simulink library "libc_control_pressure"  (R2015b)
settings: Solver=FixedStepDiscrete  StartTime=0.0  StopTime=Inf  FixedStep=0.004  RelTol=1e-3
PostLoadFcn:
  | , if any(exist('dsrtsu_mdlpostloadfcn', 'file') == [2, 3, 6]), try dsrtsu_mdlpostloadfcn('Execute', bdroot); catch fprintf('Error in PostLoadFcn (dsrtsu_mdlpostloadfcn) for model "%s":\n %s\n', bdroot, lasterr); end, end,
undefined symbols (not defined in the file or in its folder): CONST, den, DiscIntNeverNeededParam, num, p1i, tA
libraries: simulink x21, libc_parts_valves x17, libc_filters_diff x9, libbha_parts_bellows x4, libc_parts_tubes x2, PMC_lib x1
(part 1 of 2)
settings Model: DSRTSU_INTERNAL_RTI_VER=470  DSRTSU_INTERNAL_RTI_TYPE=rti1007  DSRTSU_INTERNAL_RTIFPGA=60  Creator=Falkenhahn  LastModifiedBy=Falkenhahn
settings DataIOCC: SaveFormat=Array
settings OptimizationCC: BlockReduction=off  OptimizeBlockIOStorage=off  BufferReuse=off  GlobalBufferReuse=off  ExpressionFolding=off  LocalBlockOutputs=off
settings DebuggingCC: UnderspecifiedInitializationDetection=Classic  MergeDetectMultiDrivingBlocksExec=none  SolverPrmCheckMsg=warning
settings HardwareCC: ProdBitPerPointer=32  ProdLargestAtomicFloat=None  ProdEndianess=BigEndian  ProdWordSize=32  ProdHWDeviceType=Generic->Custom  TargetIntDivRoundTo=Zero  TargetEndianess=BigEndian  TargetHWDeviceType=Generic->Custom
settings RTWCC: SystemTargetFile=rti1007.tlc  MakeCommand=make_rti  TemplateMakefile=rti1007.tmf  Description=dSPACE DS1007 Hardware Platform
settings STFCustomTargetCC: ParMdlRefBuildCompliant=on  ConcurrentExecutionCompliant=off  MatFileLogging=on  SystemTargetFile=rti1007.tlc
settings GRTTargetCC: CompOptLevelCompliant=off  ConcurrentExecutionCompliant=off  GeneratePreprocessorConditionals=Disable all  CombineOutputUpdateFcns=off  GRTInterface=on  UseToolchainInfoCompliant=off  ExtModeMexFile=noextcomm
settings ConfigComp: CovModelRefEnable=Off

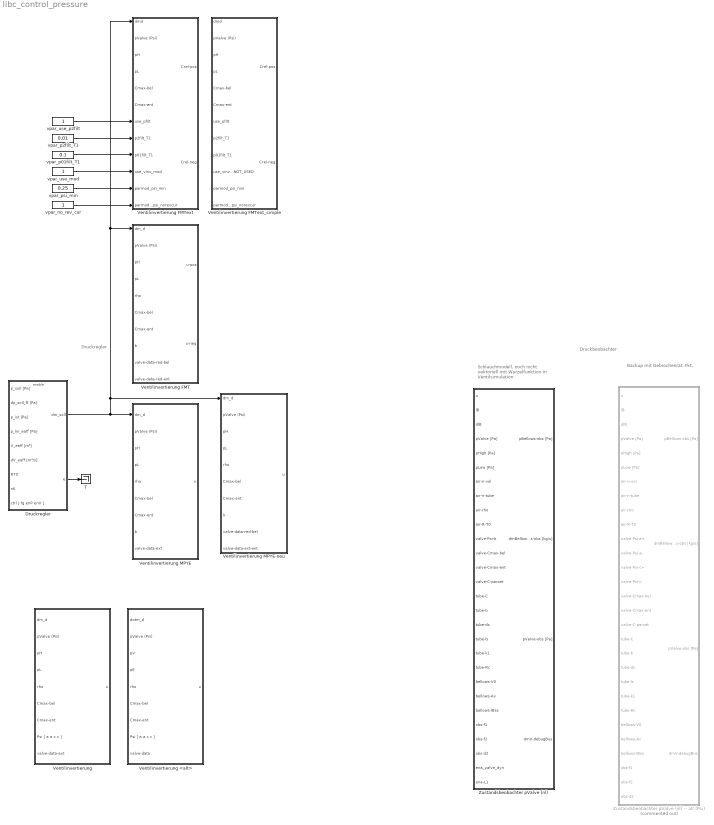
== system libc_control_pressure ==
  note: Backup mit Gebrochenrat. Fkt.
  note: Schlauchmodell, noch nicht vektoriell
      | mit Wurzelfunktion in Ventilsimulation
  note: Druckregler
  note: Druckbeobachter
  Druckregler : Subsystem
  T : Terminator
  Ventilinvertierung : Subsystem
      settings: AttributesFormatString=uses local sample time tA
  Ventilinvertierung <alt> : Subsystem
      settings: AttributesFormatString=uses local sample time tA
  Ventilinvertierung FMT : Subsystem
  Ventilinvertierung FMText : Subsystem
      settings: RTWFcnNameOpts=Use subsystem name  RTWFileNameOpts=Use function name
  Ventilinvertierung FMText_simple : Subsystem
      settings: RTWFcnNameOpts=Use subsystem name  RTWFileNameOpts=Use function name
  Ventilinvertierung MPYE : Subsystem
      settings: AttributesFormatString=uses local sample time tA
  Ventilinvertierung MPYE-neu : Subsystem
  Zustandsbeobachter pValve (nl) : Subsystem
  "Zustandsbeobachter pValve (nl) -- alt (Psi)" : Subsystem  Commented=on
  vpar_no_rev_cur : Constant
      settings: AttributesFormatString=|
      | Filterung des Kammerdrucks
      | bei FMT-Ventilen. Schnelle
      | Sprünge können eh nicht
      | kompensiert werden, da
      | Ventildynamik zu langsam
  vpar_p01filt_T1 : Constant  Value=0.1
  vpar_p2filt_T1 : Constant  Value=0.01
  vpar_psi_min : Constant  Value=0.25
  vpar_use_mod : Constant
  vpar_use_p2filt : Constant
  wires:
  Druckregler/2(e) -> T/1
  Druckregler/1(dm_soll) -> Ventilinvertierung MPYE-neu/1(dm_d), Ventilinvertierung FMT/1(dm_d), Ventilinvertierung FMText/1(dmd), Ventilinvertierung MPYE/1(dm_d)
  vpar_no_rev_cur/1 -> Ventilinvertierung FMText/12(parmod_psi_norevcur)
  vpar_psi_min/1 -> Ventilinvertierung FMText/11(parmod_psi_min)
  vpar_use_mod/1 -> Ventilinvertierung FMText/10(use_vinv_mod)
  vpar_p2filt_T1/1 -> Ventilinvertierung FMText/8(p2filt_T1)
  vpar_use_p2filt/1 -> Ventilinvertierung FMText/7(use_pfilt)
  vpar_p01filt_T1/1 -> Ventilinvertierung FMText/9(p01filt_T1)

== system libc_control_pressure/Druckregler ==
  note: Allgemeiner Druckregler (basierend auf dem
      | Druckregler von Alexander Hildebrandt | hild)
      |
      | Eingänge:
      | Drücke (alle in [Pa] absolut):
      | Solldruck, Solldruckänderung, Istdruck, Linearisierungsdruck
      | Volumen und Volumenänderung
      | Produkt RT0 und Polytropenkoeffizient nK
      | Reglerparameter ctrl
      |
      | Ausgang: Sollmassenstrom dm [kg/s] für Ventilinvertierung
  note: Funktionsbeschreibung
  note: Linearisierungsdruck p_lin_eaff kann entweder mit
      | Solldruck (zur Feedforward-Linearisierung) oder mit
      | Istdruck (zur Zustandslinearisierung) verwendet werden,
      | um Volumenänderungen dV =/= 0 zu kompensieren. Entsprechend
      | sollte dann auch die Volumenberechnung mittels Soll- oder Istgrößen geschehen
  note: Linearisierungsdruck
  note: Beschreibung der Parameter des Konfigurationseingangs ctrl
      | (*) empfohlener Wert
      |
      | fg [Hz]: Grenzfrequenz (*4Hz)
      | enP {0|1*}: aktiviere P-Regler
      | enV {0|1*}: aktiviere Vorsteuerung
  note: Reglerparameter "ctrl"
  p_soll [Pa] : Inport
  dp_soll_ff [Pa] : Inport  Port=2
  p_ist [Pa] : Inport  Port=3
  p_lin_eaff [Pa] : Inport  Port=4
  V_eaff [m³] : Inport  Port=5
  dV_eaff [m³/s] : Inport  Port=6
  RT0 : Inport  Port=7
  nK : Inport  Port=8
  ctrl [ fg enP enV ] : Inport  Port=9
  Enable : EnablePort  StatesWhenEnabling=reset
      settings: AttributesFormatString=%<StatesWhenEnabling> states\nwhen enabling
  Drucklinearsierung : Subsystem
  Folgeregler : Subsystem
  dm_soll : Outport
  e : Outport  Port=2
  wires:
  nK/1 -> Drucklinearsierung/7(nK)
  p_ist [Pa]/1 -> Folgeregler/3(p_ist)
  RT0/1 -> Drucklinearsierung/6(RT0)
  ctrl [ fg enP enV ]/1 -> Folgeregler/4(ctrl [ fgP enP enV ])
  p_lin_eaff [Pa]/1 -> Drucklinearsierung/5(p (E/A))
  dV_eaff [m³/s]/1 -> Drucklinearsierung/4(dV)
  V_eaff [m³]/1 -> Drucklinearsierung/3(V)
  Folgeregler/1(e) -> e/1
  p_soll [Pa]/1 -> Folgeregler/1(p_soll)
  dp_soll_ff [Pa]/1 -> Folgeregler/2(dp_soll)
  Folgeregler/3(nu_Vst) -> Drucklinearsierung/2(nu_in_Vorst)
  Folgeregler/2(nu_P) -> Drucklinearsierung/1(nu_in_PReg)
  Drucklinearsierung/1(dm) -> dm_soll/1

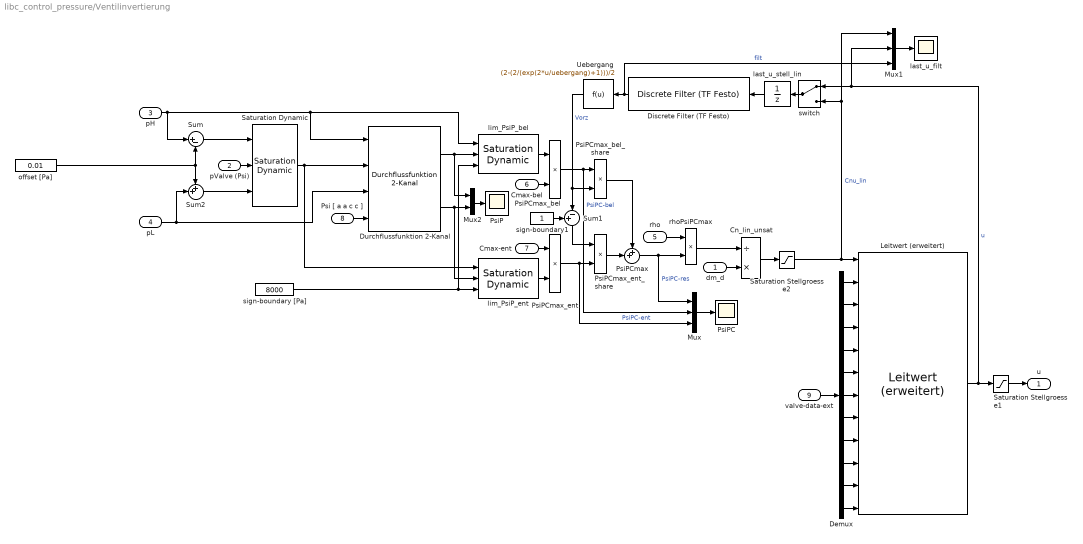
== system libc_control_pressure/Ventilinvertierung ==
  dm_d : Inport
  pValve (Psi) : Inport  Port=2
  pH : Inport  Port=3
  pL : Inport  Port=4
  rho : Inport  Port=5
  Cmax-bel : Inport  Port=6
  Cmax-ent : Inport  Port=7
  Psi [ a a c c ] : Inport  Port=8
  valve-data-ext : Inport  Port=9
  Cn_lin_unsat : Product  Inputs=/*
  Demux : Demux  Outputs=11
  Discrete Filter (TF Festo) : libc_filters_diff/Discrete Filter (TF Festo)  num_a=[1]  den_a=[1/(2*pi*3), 1]  Tsamp=tA  method='ramp'  dar='z'
      settings: AttributesFormatString=|
      | sample time: %<Tsamp> (3Hz)
      | Erhöhung der Eckfrequenz bringt keine
      | sichtbare Performanceverbesserung,
      | nur das Ventilknattern wird lauter.
  Durchflussfunktion 2-Kanal : libc_parts_valves/Durchflussfunktion 2-Kanal
      settings: AttributesFormatString=gebrochenrational
  Leitwert (erweitert) : libc_parts_valves/Leitwert (erweitert)  invertcomp=on
      settings: AttributesFormatString=|
      | inv: Cn --> u (on)
      | hin: u --> Cn (off)
      | Invertiert: %<invertcomp>
  Mux : Mux  Inputs=3
  Mux1 : Mux  Inputs=3
  Mux2 : Mux  Inputs=2
  PsiP : Scope
  PsiPC : Scope
  PsiPCmax : Sum  Inputs=++|
  PsiPCmax_bel : Product
  PsiPCmax_bel_share : Product
  PsiPCmax_ent : Product
  PsiPCmax_ent_share : Product
  Saturation Dynamic : simulink/Discontinuities/Saturation Dynamic  OutMin=[]  OutMax=[]  OutDataTypeStr=Inherit: Same as second input  OutDataType=fixdt(1, 16)  OutScaling=2^-10  DoSatur=off
  Saturation Stellgroesse1 : Saturate  UpperLimit=1  LowerLimit=-1
  Saturation Stellgroesse2 : Saturate  UpperLimit=1  LowerLimit=-1
  Sum : Sum  Inputs=|+-
  Sum1 : Sum  Inputs=+-|
  Sum2 : Sum  Inputs=++|
  Uebergang : Fcn  Expr=(2-(2/(exp(2*u/uebergang)+1)))/2  mask{uebergang=0.1}
      mask prompts: uebergang "Bereich der sanften Umschaltung"
      mask init:
      | u=-1:uebergang:1;
      | y=(tanh(u/uebergang)+1)/2;
      settings: AttributesFormatString=|
      | Weichheit des
      | Übergangs
      | testen (0.1)
      mask Display: plot(u,y)
  last_u_filt : Scope
  last_u_stell_lin : UnitDelay  SampleTime=-1
  lim_PsiP_bel : simulink/Discontinuities/Saturation Dynamic  OutMin=[]  OutMax=[]  OutDataTypeStr=Inherit: Same as second input  OutDataType=fixdt(1, 16)  OutScaling=2^-10  DoSatur=off
  lim_PsiP_ent : simulink/Discontinuities/Saturation Dynamic  OutMin=[]  OutMax=[]  OutDataTypeStr=Inherit: Same as second input  OutDataType=fixdt(1, 16)  OutScaling=2^-10  DoSatur=off
      settings: AttributesFormatString=|
      | PsiP ist immer positiv.
      | PsiP-bel wird durch Kammerdruck
      | beschränkt, nicht durch Entlüftungsdruck
  offset [Pa] : Constant  Value=0.01  SampleTime=tA
      settings: AttributesFormatString=|
      | Num. Offset
      | ca. 0.01 bar als numerische Begrenzung
      | für Psi*P in Randbereichen, damit nicht
      | gegen 0 und Cn_lin_unsat nicht viel zu groß.
      | Jetzt kleiner, da zusätzliche Begrenzung später
      | 
      | sample time: %<SampleTime>
  rhoPsiPCmax : Product  Inputs=**
  sign-boundary [Pa] : Constant  Value=8000
      settings: AttributesFormatString=|
      | untere Grenze für PsiP
      | Da diese Zahl später im Nenner stehen wird, sollte dies etwas größer
      | als 0 sein. Für den numerischen Offset hat sich ein Richtwert von 1000 Pa
      | in der Praxis (untere Grenze) bewährt. Rechnet man dies weiter, kommen
      | für Psi bei pL=1bar, pH=2bar 0.04285 und 0.08065 heraus. PsiP liegt dann bei
      | 8570 und 8146 Pa. Dies lässt sich gut mit 8000Pa abschätzen, sodass der Offset
      | wieder rein numerischer Natur (0.01) sein kann.
      | 
      | Wann wirkt dies: Bei stationären Gleichgewichtslagen (Psi ~0) am Rand des
      | Druckbereichs (nahe Versorgung oder nahe Umgebung) --> Ventil rattert
  sign-boundary1 : Constant
  switch : ManualSwitch
      settings: AttributesFormatString=|
      | da nur Vorzeichen
      | relevant ist, ist es
      | eigentlich egal, ob
      | u oder Cn(u) ver-
      | wendet wird.
      | 
      | Allerdings wirkt
      | Übergang auf u
  u : Outport
  wires:
  rho/1 -> rhoPsiPCmax/1
  Cmax-ent/1 -> PsiPCmax_ent/1
  Cmax-bel/1 -> PsiPCmax_bel/2
  Psi [ a a c c ]/1 -> Durchflussfunktion 2-Kanal/4
  valve-data-ext/1 -> Demux/1
  dm_d/1 -> Cn_lin_unsat/2
  pL/1 -> Sum2/2, Durchflussfunktion 2-Kanal/3
  pValve (Psi)/1 -> Saturation Dynamic/2
  pH/1 -> Sum/1, Durchflussfunktion 2-Kanal/1, lim_PsiP_bel/1
  Mux/1 -> PsiPC/1
  sign-boundary1/1 -> Sum1/1
  Sum1/1 -> PsiPCmax_ent_share/1
  PsiPCmax_ent/1 -> Mux/3, PsiPCmax_ent_share/2  "PsiPC-ent"
  PsiPCmax_bel/1 -> Mux/2, PsiPCmax_bel_share/1  "PsiPC-bel"
  PsiPCmax_bel_share/1 -> PsiPCmax/1
  PsiPCmax_ent_share/1 -> PsiPCmax/2
  Durchflussfunktion 2-Kanal/2 -> lim_PsiP_ent/2, Mux2/2
  Discrete Filter (TF Festo)/1 -> Uebergang/1, Mux1/3  "filt"
  rhoPsiPCmax/1 -> Cn_lin_unsat/1
  PsiPCmax/1 -> Mux/1, rhoPsiPCmax/2  "PsiPC-res"
  lim_PsiP_ent/1 -> PsiPCmax_ent/2
  lim_PsiP_bel/1 -> PsiPCmax_bel/1
  sign-boundary [Pa]/1 -> lim_PsiP_ent/3, lim_PsiP_bel/3
  switch/1 -> last_u_stell_lin/1
  Sum2/1 -> Saturation Dynamic/3
  offset [Pa]/1 -> Sum2/1, Sum/2
  Cn_lin_unsat/1 -> Saturation Stellgroesse2/1
  Durchflussfunktion 2-Kanal/1 -> lim_PsiP_bel/2, Mux2/1
  Saturation Dynamic/1 -> lim_PsiP_ent/1, Durchflussfunktion 2-Kanal/2
  Saturation Stellgroesse2/1 -> Leitwert (erweitert)/1, switch/2, Mux1/1  "Cnu_lin"
  last_u_stell_lin/1 -> Discrete Filter (TF Festo)/1
  Uebergang/1 -> Sum1/2, PsiPCmax_bel_share/2  "Vorz"
  Sum/1 -> Saturation Dynamic/1
  Leitwert (erweitert)/1 -> switch/1, Mux1/2, Saturation Stellgroesse1/1  "u"
  Demux/1 -> Leitwert (erweitert)/2
  Demux/2 -> Leitwert (erweitert)/3
  Demux/3 -> Leitwert (erweitert)/4
  Demux/4 -> Leitwert (erweitert)/5
  Demux/5 -> Leitwert (erweitert)/6
  Demux/6 -> Leitwert (erweitert)/7
  Demux/7 -> Leitwert (erweitert)/8
  Mux1/1 -> last_u_filt/1
  Mux2/1 -> PsiP/1
  Demux/11 -> Leitwert (erweitert)/12
  Demux/9 -> Leitwert (erweitert)/10
  Demux/10 -> Leitwert (erweitert)/11
  Demux/8 -> Leitwert (erweitert)/9
  Saturation Stellgroesse1/1 -> u/1

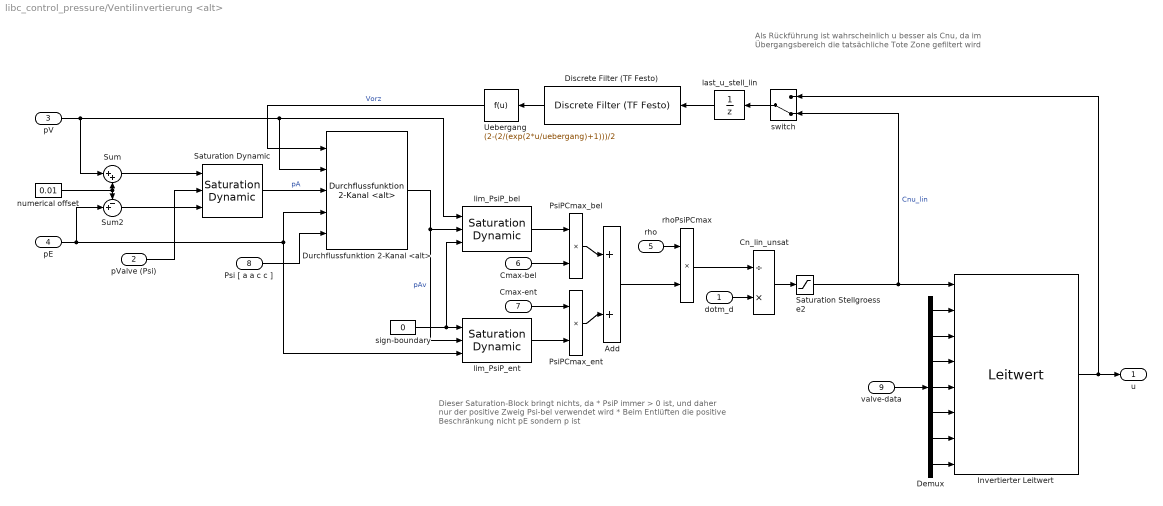
== system libc_control_pressure/Ventilinvertierung <alt> ==
  note: Dieser Saturation-Block bringt nichts, da
      | * PsiP immer > 0 ist, und daher nur der positive Zweig Psi-bel verwendet wird
      | * Beim Entlüften die positive Beschränkung nicht pE sondern p ist
  note: Als Rückführung ist wahrscheinlich u besser als Cnu, da
      | im Übergangsbereich die tatsächliche Tote Zone gefiltert wird
  dotm_d : Inport
  pValve (Psi) : Inport  Port=2
  pV : Inport  Port=3
  pE : Inport  Port=4
  rho : Inport  Port=5
  Cmax-bel : Inport  Port=6
  Cmax-ent : Inport  Port=7
  Psi [ a a c c ] : Inport  Port=8
  valve-data : Inport  Port=9
  Add : Sum  Inputs=+|+
  Cn_lin_unsat : Product  Inputs=/*
  Demux : Demux  Outputs=7
  Discrete Filter (TF Festo) : libc_filters_diff/Discrete Filter (TF Festo)  num_a=[1]  den_a=[1/(2*pi*3), 1]  Tsamp=tA  method='ramp'  dar='z'
      settings: AttributesFormatString=|
      | sample time: %<Tsamp> (3Hz)
      | Erhöhung der Eckfrequenz bringt keine
      | sichtbare Performanceverbesserung,
      | nur das Ventilknattern wird lauter.
  Durchflussfunktion 2-Kanal <alt> : libc_parts_valves/Durchflussfunktion 2-Kanal <alt>
      settings: AttributesFormatString=gebrochenrational
  Invertierter Leitwert : libc_parts_valves/Leitwert  invertcomp=on
      settings: AttributesFormatString=|
      | inv: Cn --> u (on)
      | hin: u --> Cn (off)
      | Invertiert: %<invertcomp>
  PsiPCmax_bel : Product
  PsiPCmax_ent : Product
  Saturation Dynamic : simulink/Discontinuities/Saturation Dynamic  OutMin=[]  OutMax=[]  OutDataTypeStr=Inherit: Same as second input  OutDataType=fixdt(1, 16)  OutScaling=2^-10  DoSatur=off
  Saturation Stellgroesse2 : Saturate  UpperLimit=1  LowerLimit=-1
  Sum : Sum  Inputs=|++
  Sum2 : Sum  Inputs=-+|
  Uebergang : Fcn  Expr=(2-(2/(exp(2*u/uebergang)+1)))/2  mask{uebergang=0.1}
      mask prompts: uebergang "Bereich der sanften Umschaltung"
      mask init:
      | u=-1:uebergang:1;
      | y=(tanh(u/uebergang)+1)/2;
      mask Display: plot(u,y)
  last_u_stell_lin : UnitDelay  SampleTime=-1
  lim_PsiP_bel : simulink/Discontinuities/Saturation Dynamic  OutMin=[]  OutMax=[]  OutDataTypeStr=Inherit: Same as second input  OutDataType=fixdt(1, 16)  OutScaling=2^-10  DoSatur=off
  lim_PsiP_ent : simulink/Discontinuities/Saturation Dynamic  OutMin=[]  OutMax=[]  OutDataTypeStr=Inherit: Same as second input  OutDataType=fixdt(1, 16)  OutScaling=2^-10  DoSatur=off
  numerical offset : Constant  Value=0.01  SampleTime=tA
  rhoPsiPCmax : Product  Inputs=**
  sign-boundary : Constant  Value=0
  switch : ManualSwitch  CurrentSetting=0
      settings: AttributesFormatString=|
      | da nur Vorzeichen
      | relevant ist, ist es
      | eigentlich egal, ob
      | u oder Cn(u) ver-
      | wendet wird.
  u : Outport
  wires:
  Demux/7 -> Invertierter Leitwert/8
  Demux/6 -> Invertierter Leitwert/7
  Demux/5 -> Invertierter Leitwert/6
  Demux/4 -> Invertierter Leitwert/5
  Demux/3 -> Invertierter Leitwert/4
  Demux/2 -> Invertierter Leitwert/3
  Demux/1 -> Invertierter Leitwert/2
  Invertierter Leitwert/1 -> u/1, switch/1
  Discrete Filter (TF Festo)/1 -> Uebergang/1
  pV/1 -> Durchflussfunktion 2-Kanal <alt>/2, lim_PsiP_bel/1, Sum/1
  Sum/1 -> Saturation Dynamic/1
  Uebergang/1 -> Durchflussfunktion 2-Kanal <alt>/1  "Vorz"
  last_u_stell_lin/1 -> Discrete Filter (TF Festo)/1
  pValve (Psi)/1 -> Saturation Dynamic/2
  Saturation Stellgroesse2/1 -> switch/2, Invertierter Leitwert/1  "Cnu_lin"
  Saturation Dynamic/1 -> Durchflussfunktion 2-Kanal <alt>/3  "pA"
  Durchflussfunktion 2-Kanal <alt>/1 -> lim_PsiP_ent/2, lim_PsiP_bel/2  "pAv"
  Cn_lin_unsat/1 -> Saturation Stellgroesse2/1
  pE/1 -> Sum2/2, Durchflussfunktion 2-Kanal <alt>/4, lim_PsiP_ent/3
  numerical offset/1 -> Sum2/1, Sum/2
  Sum2/1 -> Saturation Dynamic/3
  switch/1 -> last_u_stell_lin/1
  dotm_d/1 -> Cn_lin_unsat/2
  valve-data/1 -> Demux/1
  Psi [ a a c c ]/1 -> Durchflussfunktion 2-Kanal <alt>/5
  Cmax-bel/1 -> PsiPCmax_bel/2
  sign-boundary/1 -> lim_PsiP_ent/1, lim_PsiP_bel/3
  lim_PsiP_bel/1 -> PsiPCmax_bel/1
  lim_PsiP_ent/1 -> PsiPCmax_ent/2
  Cmax-ent/1 -> PsiPCmax_ent/1
  PsiPCmax_bel/1 -> Add/1
  PsiPCmax_ent/1 -> Add/2
  Add/1 -> rhoPsiPCmax/2
  rho/1 -> rhoPsiPCmax/1
  rhoPsiPCmax/1 -> Cn_lin_unsat/1

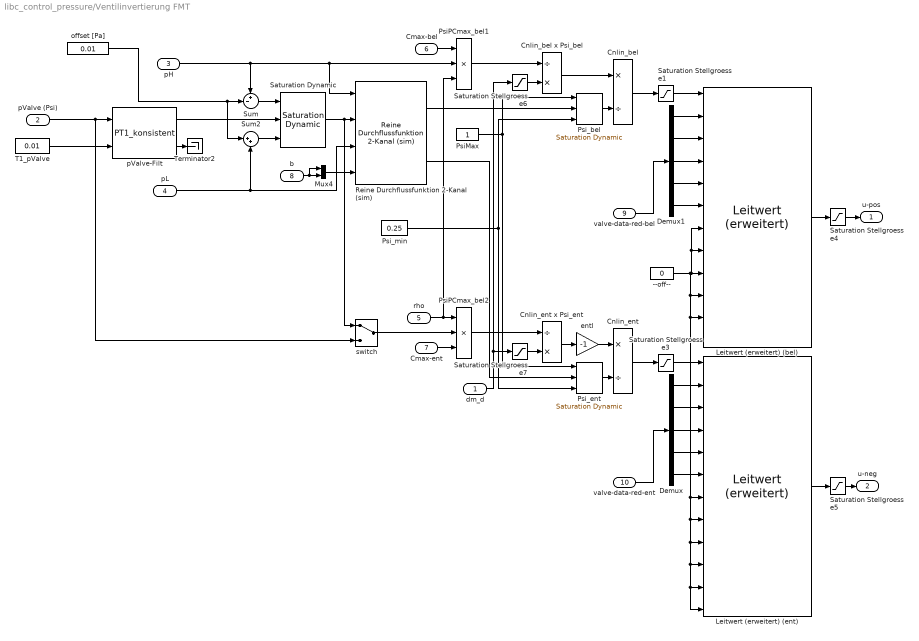
== system libc_control_pressure/Ventilinvertierung FMT ==
  dm_d : Inport
  pValve (Psi) : Inport  Port=2
  pH : Inport  Port=3
  pL : Inport  Port=4
  rho : Inport  Port=5
  Cmax-bel : Inport  Port=6
  Cmax-ent : Inport  Port=7
  b : Inport  Port=8
  valve-data-red-bel : Inport  Port=9
  valve-data-red-ent : Inport  Port=10
  --off-- : Constant  Value=0
  Cnlin_bel : Product  Inputs=*/
  Cnlin_bel x Psi_bel : Product  Inputs=/*
  Cnlin_ent : Product  Inputs=*/
  Cnlin_ent x Psi_ent : Product  Inputs=/*
  Demux : Demux  Outputs=5
  Demux1 : Demux  Outputs=5
  Leitwert (erweitert) (bel) : libc_parts_valves/Leitwert (erweitert)  invertcomp=on
      settings: AttributesFormatString=|
      | inv: Cn --> u (on)
      | hin: u --> Cn (off)
      | Invertiert: %<invertcomp>
  Leitwert (erweitert) (ent) : libc_parts_valves/Leitwert (erweitert)  invertcomp=on
      settings: AttributesFormatString=|
      | inv: Cn --> u (on)
      | hin: u --> Cn (off)
      | Invertiert: %<invertcomp>
  Mux4 : Mux  Inputs=2
  PsiMax : Constant
  PsiPCmax_bel1 : Product  Inputs=3
  PsiPCmax_bel2 : Product  Inputs=3
  Psi_bel : simulink/Discontinuities/Saturation Dynamic  OutMin=[]  OutMax=[]  OutDataTypeStr=Inherit: Same as second input  OutDataType=fixdt(1, 16)  OutScaling=2^-10  DoSatur=off
      settings: AttributesFormatString=|
      | Psi sollte nicht zu klein werden,
      | sonst wird die Verstärkung aufgrund eines
      | Druckverhältnisses nahe 1 zu stark
  Psi_ent : simulink/Discontinuities/Saturation Dynamic  OutMin=[]  OutMax=[]  OutDataTypeStr=Inherit: Same as second input  OutDataType=fixdt(1, 16)  OutScaling=2^-10  DoSatur=off
      settings: AttributesFormatString=|
      | Psi sollte nicht zu klein werden,
      | sonst wird die Verstärkung aufgrund eines
      | Druckverhältnisses nahe 1 zu stark
  Psi_min : Constant  Value=0.25
      settings: AttributesFormatString=|
      | je nach Anwendung
      | zwischen 0.1 und 0.25
      | (max. Verstärkung durch
      | schlechtes Druckverhältnis
      | zwischen 10 und 4)
  Reine Durchflussfunktion 2-Kanal (sim) : libc_parts_valves/Reine Durchflussfunktion 2-Kanal (sim)
      settings: AttributesFormatString=Wurzelfunktion
  Saturation Dynamic : simulink/Discontinuities/Saturation Dynamic  OutMin=[]  OutMax=[]  OutDataTypeStr=Inherit: Same as second input  OutDataType=fixdt(1, 16)  OutScaling=2^-10  DoSatur=off
  Saturation Stellgroesse{1,3..5} (4 alike) : Saturate  UpperLimit=1  LowerLimit=0
  Saturation Stellgroesse6 : Saturate  UpperLimit=inf  LowerLimit=0
  Saturation Stellgroesse7 : Saturate  UpperLimit=0  LowerLimit=-inf
  Sum : Sum  Inputs=+-|
  Sum2 : Sum  Inputs=|++
  T1_pValve : Constant  Value=0.01
      settings: AttributesFormatString=|
      | Filterung des Kammerdrucks
      | bei FMT-Ventilen. Schnelle
      | Sprünge können eh nicht
      | kompensiert werden, da
      | Ventildynamik zu langsam
  Terminator2 : Terminator
  entl : Gain  Gain=-1
  offset [Pa] : Constant  Value=0.01  SampleTime=tA
      settings: AttributesFormatString=|
      | Num. Offset
      | ca. 0.01 Pa als numerische Begrenzung, dass
      | Ventildruck immer innerhalb der Druckbegrenzung
      | 
      | sample time: %<SampleTime>
  pValve-Filt : libc_filters_diff/PT1_konsistent
  switch : ManualSwitch
      settings: AttributesFormatString=|
      | Treibender Druck
      | gesättigt/gefiltert
      | oder nicht?
  u-pos : Outport
  u-neg : Outport  Port=2
  wires:
  --off--/1 -> Leitwert (erweitert) (ent)/12, Leitwert (erweitert) (ent)/11, Leitwert (erweitert) (ent)/10, Leitwert (erweitert) (ent)/9, Leitwert (erweitert) (ent)/8, Leitwert (erweitert) (ent)/7, Leitwert (erweitert) (bel)/12, Leitwert (erweitert) (bel)/11, Leitwert (erweitert) (bel)/10, Leitwert (erweitert) (bel)/7, Leitwert (erweitert) (bel)/8, Leitwert (erweitert) (bel)/9
  Leitwert (erweitert) (ent)/1 -> Saturation Stellgroesse5/1
  Psi_min/1 -> Psi_ent/3, Psi_bel/3
  PsiMax/1 -> Psi_bel/1, Psi_ent/1
  Mux4/1 -> Reine Durchflussfunktion 2-Kanal (sim)/4
  b/1 -> Mux4/2, Mux4/1
  Reine Durchflussfunktion 2-Kanal (sim)/1 -> Psi_bel/2
  Reine Durchflussfunktion 2-Kanal (sim)/2 -> Psi_ent/2
  Cmax-ent/1 -> PsiPCmax_bel2/3
  Cmax-bel/1 -> PsiPCmax_bel1/1
  rho/1 -> PsiPCmax_bel2/1, PsiPCmax_bel1/3
  dm_d/1 -> Saturation Stellgroesse7/1, Saturation Stellgroesse6/1
  entl/1 -> Cnlin_ent/1
  Psi_ent/1 -> Cnlin_ent/2
  Cnlin_ent x Psi_ent/1 -> entl/1
  Psi_bel/1 -> Cnlin_bel/2
  Cnlin_bel x Psi_bel/1 -> Cnlin_bel/1
  PsiPCmax_bel2/1 -> Cnlin_ent x Psi_ent/1
  PsiPCmax_bel1/1 -> Cnlin_bel x Psi_bel/1
  Saturation Stellgroesse6/1 -> Cnlin_bel x Psi_bel/2
  pValve-Filt/1 -> Saturation Dynamic/2
  T1_pValve/1 -> pValve-Filt/2
  pValve-Filt/2 -> Terminator2/1
  pValve (Psi)/1 -> switch/2, pValve-Filt/1
  Cnlin_ent/1 -> Saturation Stellgroesse3/1
  Cnlin_bel/1 -> Saturation Stellgroesse1/1
  Saturation Stellgroesse7/1 -> Cnlin_ent x Psi_ent/2
  valve-data-red-ent/1 -> Demux/1
  valve-data-red-bel/1 -> Demux1/1
  Demux1/5 -> Leitwert (erweitert) (bel)/6
  Demux1/4 -> Leitwert (erweitert) (bel)/5
  Demux1/3 -> Leitwert (erweitert) (bel)/4
  Demux1/2 -> Leitwert (erweitert) (bel)/3
  Demux1/1 -> Leitwert (erweitert) (bel)/2
  Demux/5 -> Leitwert (erweitert) (ent)/6
  Demux/4 -> Leitwert (erweitert) (ent)/5
  Demux/3 -> Leitwert (erweitert) (ent)/4
  Demux/2 -> Leitwert (erweitert) (ent)/3
  Demux/1 -> Leitwert (erweitert) (ent)/2
  Leitwert (erweitert) (bel)/1 -> Saturation Stellgroesse4/1
  Saturation Stellgroesse5/1 -> u-neg/1
  Saturation Stellgroesse4/1 -> u-pos/1
  Saturation Stellgroesse1/1 -> Leitwert (erweitert) (bel)/1
  Saturation Stellgroesse3/1 -> Leitwert (erweitert) (ent)/1
  pL/1 -> Reine Durchflussfunktion 2-Kanal (sim)/3, Sum2/2
  Saturation Dynamic/1 -> switch/1, Reine Durchflussfunktion 2-Kanal (sim)/2
  pH/1 -> Sum/1, PsiPCmax_bel1/2, Reine Durchflussfunktion 2-Kanal (sim)/1
  Sum/1 -> Saturation Dynamic/1
  Sum2/1 -> Saturation Dynamic/3
  offset [Pa]/1 -> Sum2/1, Sum/2
  switch/1 -> PsiPCmax_bel2/2

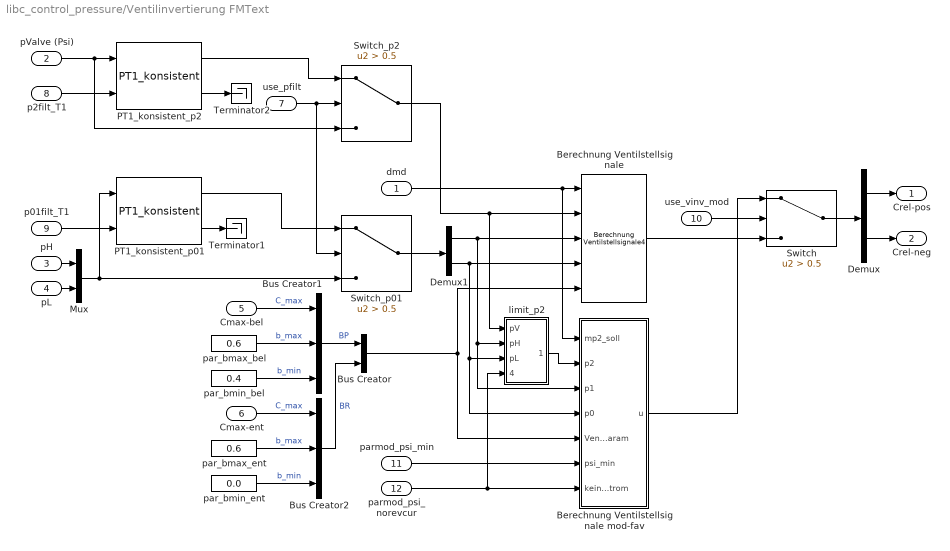
== system libc_control_pressure/Ventilinvertierung FMText ==
  dmd : Inport
  pValve (Psi) : Inport  Port=2
  pH : Inport  Port=3
  pL : Inport  Port=4
  Cmax-bel : Inport  Port=5
  Cmax-ent : Inport  Port=6
  use_pfilt : Inport  Port=7
  p2filt_T1 : Inport  Port=8
  p01filt_T1 : Inport  Port=9
  use_vinv_mod : Inport  Port=10
  parmod_psi_min : Inport  Port=11
  parmod_psi_norevcur : Inport  Port=12
  Berechnung Ventilstellsignale : PMC_lib/Massenstrom 2 Boosterhub/Berechnung Ventilstellsignale4
  Berechnung Ventilstellsignale mod-fav : Subsystem
      mask help: Umrechnung eines gewünschten Massenstroms in ein entsprechendes Ventilstellsignal unter Verwendung der inversen Ventilkennlinie.
      settings: RTWFcnNameOpts=Use subsystem name  RTWFileNameOpts=Use subsystem name
      settings: AttributesFormatString=|
      | modifizierte Ventilkennlinie
      | mit Begrenzung von Psi
      | (e.g. >=0.25) und
      | pValve in [pL,pH]
  Bus Creator : BusCreator  Inputs=2
  Bus Creator1 : BusCreator  Inputs=3
  Bus Creator2 : BusCreator  Inputs=3
  Demux : Demux  Outputs=2
  Demux1 : Demux  Outputs=2
  Mux : Mux  Inputs=2
  PT1_konsistent_p01 : libc_filters_diff/PT1_konsistent
  PT1_konsistent_p2 : libc_filters_diff/PT1_konsistent
  Switch : Switch  Criteria=u2 > Threshold  Threshold=0.5
  Switch_p01 : Switch  Criteria=u2 > Threshold  Threshold=0.5
  Switch_p2 : Switch  Criteria=u2 > Threshold  Threshold=0.5
  Terminator1 : Terminator
  Terminator2 : Terminator
  limit_p2 : Subsystem
  par_bmax_bel : Constant  Value=0.6
  par_bmax_ent : Constant  Value=0.6
  par_bmin_bel : Constant  Value=0.4
  par_bmin_ent : Constant  Value=0.0
  Crel-pos : Outport
  Crel-neg : Outport  Port=2
  wires:
  use_vinv_mod/1 -> Switch/2
  p2filt_T1/1 -> PT1_konsistent_p2/2
  use_pfilt/1 -> Switch_p01/2, Switch_p2/2
  pValve (Psi)/1 -> PT1_konsistent_p2/1, Switch_p2/3
  PT1_konsistent_p2/2 -> Terminator2/1
  PT1_konsistent_p2/1 -> Switch_p2/1
  Berechnung Ventilstellsignale mod-fav/1(u) -> Switch/1
  Switch/1 -> Demux/1
  Berechnung Ventilstellsignale/1 -> Switch/3
  parmod_psi_norevcur/1 -> Berechnung Ventilstellsignale mod-fav/7(kein_rueckstrom), limit_p2/4(limit)
  parmod_psi_min/1 -> Berechnung Ventilstellsignale mod-fav/6(psi_min)
  Demux1/2 -> Berechnung Ventilstellsignale/4, limit_p2/3(pL), Berechnung Ventilstellsignale mod-fav/4(p0)
  Demux1/1 -> limit_p2/2(pH), Berechnung Ventilstellsignale mod-fav/3(p1), Berechnung Ventilstellsignale/3
  Switch_p2/1 -> Berechnung Ventilstellsignale/2, limit_p2/1(pV)
  dmd/1 -> Berechnung Ventilstellsignale/1, Berechnung Ventilstellsignale mod-fav/1(mp2_soll)
  par_bmin_ent/1 -> Bus Creator2/3  "b_min"
  par_bmax_ent/1 -> Bus Creator2/2  "b_max"
  Cmax-ent/1 -> Bus Creator2/1  "C_max"
  par_bmin_bel/1 -> Bus Creator1/3  "b_min"
  Cmax-bel/1 -> Bus Creator1/1  "C_max"
  par_bmax_bel/1 -> Bus Creator1/2  "b_max"
  Bus Creator2/1 -> Bus Creator/2  "BR"
  Bus Creator1/1 -> Bus Creator/1  "BP"
  Bus Creator/1 -> Berechnung Ventilstellsignale/5, Berechnung Ventilstellsignale mod-fav/5(Ventilparam)
  Demux/2 -> Crel-neg/1
  Demux/1 -> Crel-pos/1
  pH/1 -> Mux/1
  pL/1 -> Mux/2
  Switch_p01/1 -> Demux1/1
  Mux/1 -> PT1_konsistent_p01/1, Switch_p01/3
  PT1_konsistent_p01/2 -> Terminator1/1
  PT1_konsistent_p01/1 -> Switch_p01/1
  p01filt_T1/1 -> PT1_konsistent_p01/2
  limit_p2/1(pVlim) -> Berechnung Ventilstellsignale mod-fav/2(p2)

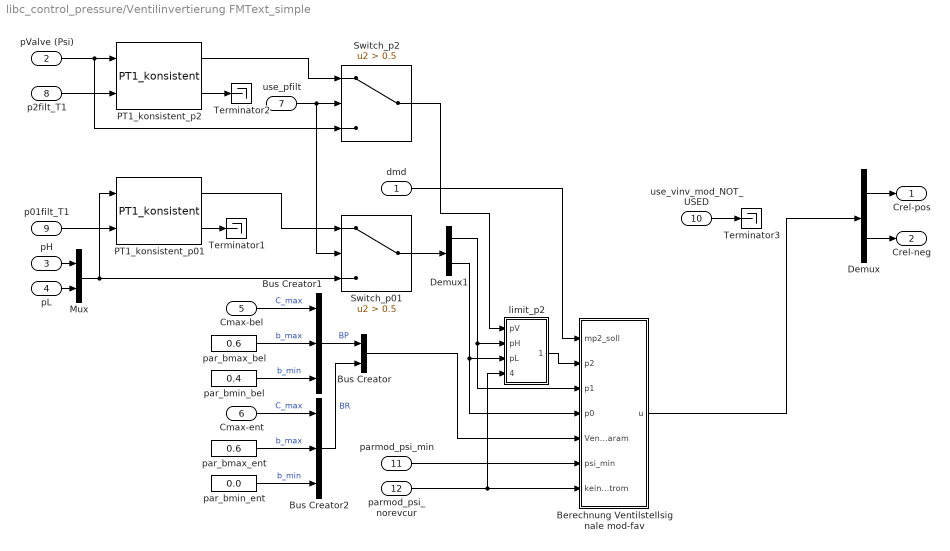
== system libc_control_pressure/Ventilinvertierung FMText_simple ==
  dmd : Inport
  pValve (Psi) : Inport  Port=2
  pH : Inport  Port=3
  pL : Inport  Port=4
  Cmax-bel : Inport  Port=5
  Cmax-ent : Inport  Port=6
  use_pfilt : Inport  Port=7
  p2filt_T1 : Inport  Port=8
  p01filt_T1 : Inport  Port=9
  use_vinv_mod_NOT_USED : Inport  Port=10
  parmod_psi_min : Inport  Port=11
  parmod_psi_norevcur : Inport  Port=12
  Berechnung Ventilstellsignale mod-fav : Subsystem
      mask help: Umrechnung eines gewünschten Massenstroms in ein entsprechendes Ventilstellsignal unter Verwendung der inversen Ventilkennlinie.
      settings: RTWFcnNameOpts=Use subsystem name  RTWFileNameOpts=Use subsystem name
      settings: AttributesFormatString=|
      | modifizierte Ventilkennlinie
      | mit Begrenzung von Psi
      | (e.g. >=0.25) und
      | pValve in [pL,pH]
  Bus Creator : BusCreator  Inputs=2
  Bus Creator1 : BusCreator  Inputs=3
  Bus Creator2 : BusCreator  Inputs=3
  Demux : Demux  Outputs=2
  Demux1 : Demux  Outputs=2
  Mux : Mux  Inputs=2
  PT1_konsistent_p01 : libc_filters_diff/PT1_konsistent
  PT1_konsistent_p2 : libc_filters_diff/PT1_konsistent
  Switch_p01 : Switch  Criteria=u2 > Threshold  Threshold=0.5
  Switch_p2 : Switch  Criteria=u2 > Threshold  Threshold=0.5
  Terminator1 : Terminator
  Terminator2 : Terminator
  Terminator3 : Terminator
  limit_p2 : Subsystem
  par_bmax_bel : Constant  Value=0.6
  par_bmax_ent : Constant  Value=0.6
  par_bmin_bel : Constant  Value=0.4
  par_bmin_ent : Constant  Value=0.0
  Crel-pos : Outport
  Crel-neg : Outport  Port=2
  wires:
  limit_p2/1(pVlim) -> Berechnung Ventilstellsignale mod-fav/2(p2)
  p01filt_T1/1 -> PT1_konsistent_p01/2
  PT1_konsistent_p01/1 -> Switch_p01/1
  PT1_konsistent_p01/2 -> Terminator1/1
  Mux/1 -> Switch_p01/3, PT1_konsistent_p01/1
  Switch_p01/1 -> Demux1/1
  pL/1 -> Mux/2
  pH/1 -> Mux/1
  Demux/1 -> Crel-pos/1
  Demux/2 -> Crel-neg/1
  Bus Creator/1 -> Berechnung Ventilstellsignale mod-fav/5(Ventilparam)
  Bus Creator1/1 -> Bus Creator/1  "BP"
  Bus Creator2/1 -> Bus Creator/2  "BR"
  par_bmax_bel/1 -> Bus Creator1/2  "b_max"
  Cmax-bel/1 -> Bus Creator1/1  "C_max"
  par_bmin_bel/1 -> Bus Creator1/3  "b_min"
  Cmax-ent/1 -> Bus Creator2/1  "C_max"
  par_bmax_ent/1 -> Bus Creator2/2  "b_max"
  par_bmin_ent/1 -> Bus Creator2/3  "b_min"
  dmd/1 -> Berechnung Ventilstellsignale mod-fav/1(mp2_soll)
  Switch_p2/1 -> limit_p2/1(pV)
  Demux1/1 -> Berechnung Ventilstellsignale mod-fav/3(p1), limit_p2/2(pH)
  Demux1/2 -> Berechnung Ventilstellsignale mod-fav/4(p0), limit_p2/3(pL)
  parmod_psi_min/1 -> Berechnung Ventilstellsignale mod-fav/6(psi_min)
  parmod_psi_norevcur/1 -> limit_p2/4(limit), Berechnung Ventilstellsignale mod-fav/7(kein_rueckstrom)
  Berechnung Ventilstellsignale mod-fav/1(u) -> Demux/1
  PT1_konsistent_p2/1 -> Switch_p2/1
  PT1_konsistent_p2/2 -> Terminator2/1
  pValve (Psi)/1 -> Switch_p2/3, PT1_konsistent_p2/1
  use_pfilt/1 -> Switch_p2/2, Switch_p01/2
  p2filt_T1/1 -> PT1_konsistent_p2/2
  use_vinv_mod_NOT_USED/1 -> Terminator3/1

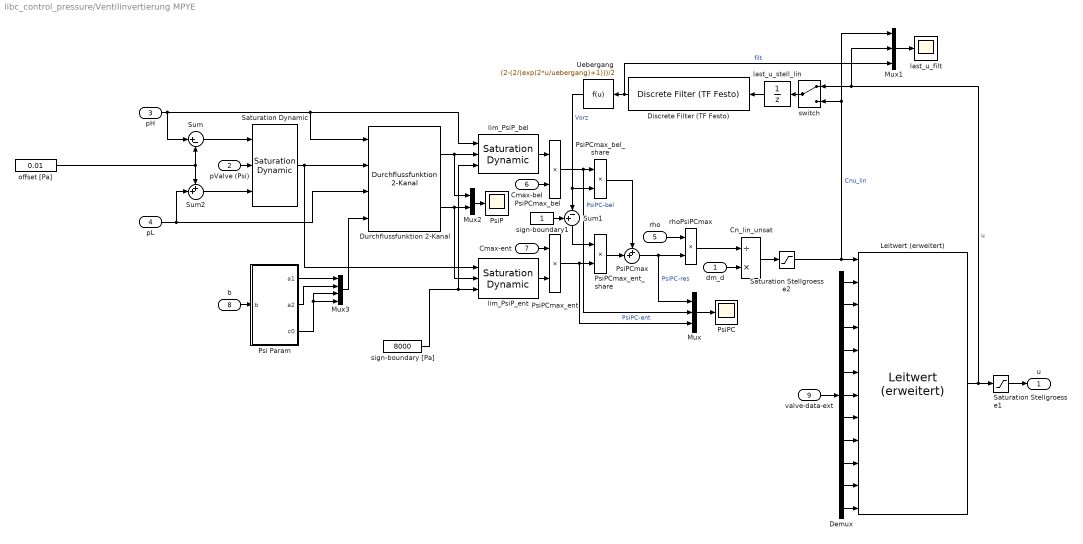
== system libc_control_pressure/Ventilinvertierung MPYE ==
  dm_d : Inport
  pValve (Psi) : Inport  Port=2
  pH : Inport  Port=3
  pL : Inport  Port=4
  rho : Inport  Port=5
  Cmax-bel : Inport  Port=6
  Cmax-ent : Inport  Port=7
  b : Inport  Port=8
  valve-data-ext : Inport  Port=9
  Cn_lin_unsat : Product  Inputs=/*
  Demux : Demux  Outputs=11
  Discrete Filter (TF Festo) : libc_filters_diff/Discrete Filter (TF Festo)  num_a=[1]  den_a=[1/(2*pi*3), 1]  Tsamp=tA  method='ramp'  dar='z'
      settings: AttributesFormatString=|
      | sample time: %<Tsamp> (3Hz)
      | Erhöhung der Eckfrequenz bringt keine
      | sichtbare Performanceverbesserung,
      | nur das Ventilknattern wird lauter.
  Durchflussfunktion 2-Kanal : libc_parts_valves/Durchflussfunktion 2-Kanal
      settings: AttributesFormatString=gebrochenrational
  Leitwert (erweitert) : libc_parts_valves/Leitwert (erweitert)  invertcomp=on
      settings: AttributesFormatString=|
      | inv: Cn --> u (on)
      | hin: u --> Cn (off)
      | Invertiert: %<invertcomp>
  Mux : Mux  Inputs=3
  Mux1 : Mux  Inputs=3
  Mux2 : Mux  Inputs=2
  Mux3 : Mux
  Psi Param : Subsystem
      settings: AttributesFormatString=sqrt -> geb-rat
  PsiP : Scope
  PsiPC : Scope
  PsiPCmax : Sum  Inputs=++|
  PsiPCmax_bel : Product
  PsiPCmax_bel_share : Product
  PsiPCmax_ent : Product
  PsiPCmax_ent_share : Product
  Saturation Dynamic : simulink/Discontinuities/Saturation Dynamic  OutMin=[]  OutMax=[]  OutDataTypeStr=Inherit: Same as second input  OutDataType=fixdt(1, 16)  OutScaling=2^-10  DoSatur=off
  Saturation Stellgroesse1 : Saturate  UpperLimit=1  LowerLimit=-1
  Saturation Stellgroesse2 : Saturate  UpperLimit=1  LowerLimit=-1
  Sum : Sum  Inputs=|+-
  Sum1 : Sum  Inputs=+-|
  Sum2 : Sum  Inputs=++|
  Uebergang : Fcn  Expr=(2-(2/(exp(2*u/uebergang)+1)))/2  mask{uebergang=0.1}
      mask prompts: uebergang "Bereich der sanften Umschaltung"
      mask init:
      | u=-1:uebergang:1;
      | y=(tanh(u/uebergang)+1)/2;
      settings: AttributesFormatString=|
      | Weichheit des
      | Übergangs
      | testen (0.1)
      mask Display: plot(u,y)
  last_u_filt : Scope
  last_u_stell_lin : UnitDelay  SampleTime=-1
  lim_PsiP_bel : simulink/Discontinuities/Saturation Dynamic  OutMin=[]  OutMax=[]  OutDataTypeStr=Inherit: Same as second input  OutDataType=fixdt(1, 16)  OutScaling=2^-10  DoSatur=off
  lim_PsiP_ent : simulink/Discontinuities/Saturation Dynamic  OutMin=[]  OutMax=[]  OutDataTypeStr=Inherit: Same as second input  OutDataType=fixdt(1, 16)  OutScaling=2^-10  DoSatur=off
      settings: AttributesFormatString=|
      | PsiP ist immer positiv.
      | PsiP-bel wird durch Kammerdruck
      | beschränkt, nicht durch Entlüftungsdruck
  offset [Pa] : Constant  Value=0.01  SampleTime=tA
      settings: AttributesFormatString=|
      | Num. Offset
      | ca. 0.01 bar als numerische Begrenzung
      | für Psi*P in Randbereichen, damit nicht
      | gegen 0 und Cn_lin_unsat nicht viel zu groß.
      | Jetzt kleiner, da zusätzliche Begrenzung später
      | 
      | sample time: %<SampleTime>
  rhoPsiPCmax : Product  Inputs=**
  sign-boundary [Pa] : Constant  Value=8000
      settings: AttributesFormatString=|
      | untere Grenze für PsiP
      | Da diese Zahl später im Nenner stehen wird, sollte dies etwas größer
      | als 0 sein. Für den numerischen Offset hat sich ein Richtwert von 1000 Pa
      | in der Praxis (untere Grenze) bewährt. Rechnet man dies weiter, kommen
      | für Psi bei pL=1bar, pH=2bar 0.04285 und 0.08065 heraus. PsiP liegt dann bei
      | 8570 und 8146 Pa. Dies lässt sich gut mit 8000Pa abschätzen, sodass der Offset
      | wieder rein numerischer Natur (0.01) sein kann.
      | 
      | Wann wirkt dies: Bei stationären Gleichgewichtslagen (Psi ~0) am Rand des
      | Druckbereichs (nahe Versorgung oder nahe Umgebung) --> Ventil rattert
  sign-boundary1 : Constant
  switch : ManualSwitch
      settings: AttributesFormatString=|
      | da nur Vorzeichen
      | relevant ist, ist es
      | eigentlich egal, ob
      | u oder Cn(u) ver-
      | wendet wird.
      | 
      | Allerdings wirkt
      | Übergang auf u
  u : Outport
  wires:
  Saturation Stellgroesse1/1 -> u/1
  Demux/8 -> Leitwert (erweitert)/9
  Demux/10 -> Leitwert (erweitert)/11
  Demux/9 -> Leitwert (erweitert)/10
  Demux/11 -> Leitwert (erweitert)/12
  Mux2/1 -> PsiP/1
  Mux1/1 -> last_u_filt/1
  Demux/7 -> Leitwert (erweitert)/8
  Demux/6 -> Leitwert (erweitert)/7
  Demux/5 -> Leitwert (erweitert)/6
  Demux/4 -> Leitwert (erweitert)/5
  Demux/3 -> Leitwert (erweitert)/4
  Demux/2 -> Leitwert (erweitert)/3
  Demux/1 -> Leitwert (erweitert)/2
  Leitwert (erweitert)/1 -> Saturation Stellgroesse1/1, Mux1/2, switch/1  "u"
  Sum/1 -> Saturation Dynamic/1
  Uebergang/1 -> PsiPCmax_bel_share/2, Sum1/2  "Vorz"
  last_u_stell_lin/1 -> Discrete Filter (TF Festo)/1
  Saturation Stellgroesse2/1 -> Mux1/1, switch/2, Leitwert (erweitert)/1  "Cnu_lin"
  Saturation Dynamic/1 -> Durchflussfunktion 2-Kanal/2, lim_PsiP_ent/1
  Durchflussfunktion 2-Kanal/1 -> Mux2/1, lim_PsiP_bel/2
  Cn_lin_unsat/1 -> Saturation Stellgroesse2/1
  offset [Pa]/1 -> Sum/2, Sum2/1
  Sum2/1 -> Saturation Dynamic/3
  switch/1 -> last_u_stell_lin/1
  sign-boundary [Pa]/1 -> lim_PsiP_bel/3, lim_PsiP_ent/3
  lim_PsiP_bel/1 -> PsiPCmax_bel/1
  lim_PsiP_ent/1 -> PsiPCmax_ent/2
  PsiPCmax/1 -> rhoPsiPCmax/2, Mux/1  "PsiPC-res"
  rhoPsiPCmax/1 -> Cn_lin_unsat/1
  Discrete Filter (TF Festo)/1 -> Mux1/3, Uebergang/1  "filt"
  Durchflussfunktion 2-Kanal/2 -> Mux2/2, lim_PsiP_ent/2
  PsiPCmax_ent_share/1 -> PsiPCmax/2
  PsiPCmax_bel_share/1 -> PsiPCmax/1
  PsiPCmax_bel/1 -> PsiPCmax_bel_share/1, Mux/2  "PsiPC-bel"
  PsiPCmax_ent/1 -> PsiPCmax_ent_share/2, Mux/3  "PsiPC-ent"
  Sum1/1 -> PsiPCmax_ent_share/1
  sign-boundary1/1 -> Sum1/1
  Mux/1 -> PsiPC/1
  pH/1 -> lim_PsiP_bel/1, Durchflussfunktion 2-Kanal/1, Sum/1
  pValve (Psi)/1 -> Saturation Dynamic/2
  pL/1 -> Durchflussfunktion 2-Kanal/3, Sum2/2
  dm_d/1 -> Cn_lin_unsat/2
  valve-data-ext/1 -> Demux/1
  Mux3/1 -> Durchflussfunktion 2-Kanal/4
  Cmax-bel/1 -> PsiPCmax_bel/2
  Cmax-ent/1 -> PsiPCmax_ent/1
  rho/1 -> rhoPsiPCmax/1
  Psi Param/3(c0) -> Mux3/4, Mux3/3
  Psi Param/2(a2) -> Mux3/2
  Psi Param/1(a1) -> Mux3/1
  b/1 -> Psi Param/1(b)

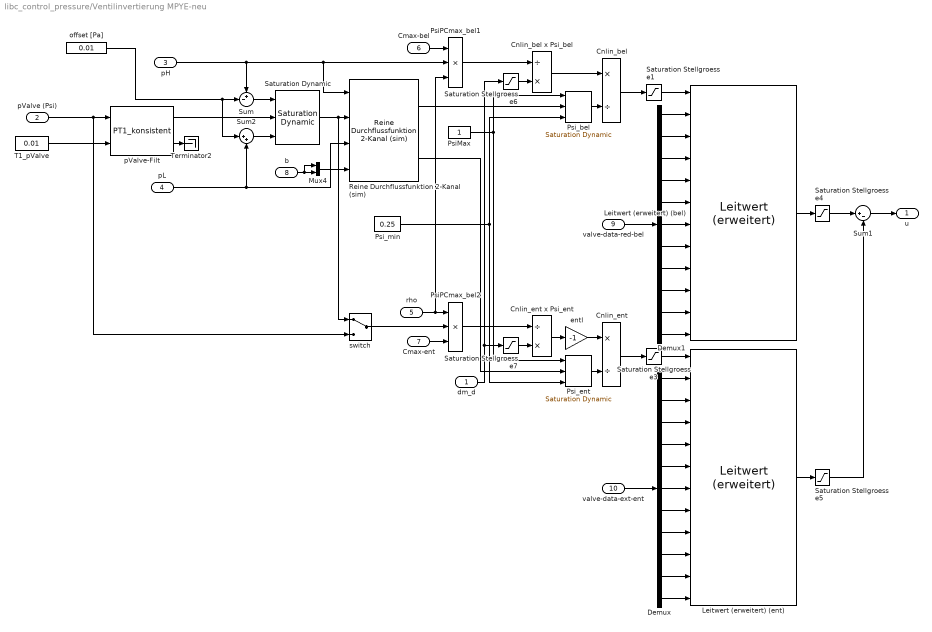
== system libc_control_pressure/Ventilinvertierung MPYE-neu ==
  dm_d : Inport
  pValve (Psi) : Inport  Port=2
  pH : Inport  Port=3
  pL : Inport  Port=4
  rho : Inport  Port=5
  Cmax-bel : Inport  Port=6
  Cmax-ent : Inport  Port=7
  b : Inport  Port=8
  valve-data-red-bel : Inport  Port=9
  valve-data-ext-ent : Inport  Port=10
  Cnlin_bel : Product  Inputs=*/
  Cnlin_bel x Psi_bel : Product  Inputs=/*
  Cnlin_ent : Product  Inputs=*/
  Cnlin_ent x Psi_ent : Product  Inputs=/*
  Demux : Demux  Outputs=11
  Demux1 : Demux  Outputs=11
  Leitwert (erweitert) (bel) : libc_parts_valves/Leitwert (erweitert)  invertcomp=on
      settings: AttributesFormatString=|
      | inv: Cn --> u (on)
      | hin: u --> Cn (off)
      | Invertiert: %<invertcomp>
  Leitwert (erweitert) (ent) : libc_parts_valves/Leitwert (erweitert)  invertcomp=on
      settings: AttributesFormatString=|
      | inv: Cn --> u (on)
      | hin: u --> Cn (off)
      | Invertiert: %<invertcomp>
  Mux4 : Mux  Inputs=2
  PsiMax : Constant
  PsiPCmax_bel1 : Product  Inputs=3
  PsiPCmax_bel2 : Product  Inputs=3
  Psi_bel : simulink/Discontinuities/Saturation Dynamic  OutMin=[]  OutMax=[]  OutDataTypeStr=Inherit: Same as second input  OutDataType=fixdt(1, 16)  OutScaling=2^-10  DoSatur=off
      settings: AttributesFormatString=|
      | Psi sollte nicht zu klein werden,
      | sonst wird die Verstärkung aufgrund eines
      | Druckverhältnisses nahe 1 zu stark
  Psi_ent : simulink/Discontinuities/Saturation Dynamic  OutMin=[]  OutMax=[]  OutDataTypeStr=Inherit: Same as second input  OutDataType=fixdt(1, 16)  OutScaling=2^-10  DoSatur=off
      settings: AttributesFormatString=|
      | Psi sollte nicht zu klein werden,
      | sonst wird die Verstärkung aufgrund eines
      | Druckverhältnisses nahe 1 zu stark
  Psi_min : Constant  Value=0.25
      settings: AttributesFormatString=|
      | je nach Anwendung
      | zwischen 0.1 und 0.25
      | (max. Verstärkung durch
      | schlechtes Druckverhältnis
      | zwischen 10 und 4)
  Reine Durchflussfunktion 2-Kanal (sim) : libc_parts_valves/Reine Durchflussfunktion 2-Kanal (sim)
      settings: AttributesFormatString=Wurzelfunktion
  Saturation Dynamic : simulink/Discontinuities/Saturation Dynamic  OutMin=[]  OutMax=[]  OutDataTypeStr=Inherit: Same as second input  OutDataType=fixdt(1, 16)  OutScaling=2^-10  DoSatur=off
  Saturation Stellgroesse{1,3..5} (4 alike) : Saturate  UpperLimit=1  LowerLimit=0
  Saturation Stellgroesse6 : Saturate  UpperLimit=inf  LowerLimit=0
  Saturation Stellgroesse7 : Saturate  UpperLimit=0  LowerLimit=-inf
  Sum : Sum  Inputs=+-|
  Sum1 : Sum  Inputs=|+-
  Sum2 : Sum  Inputs=|++
  T1_pValve : Constant  Value=0.01
      settings: AttributesFormatString=|
      | Filterung des Kammerdrucks
      | bei FMT-Ventilen. Schnelle
      | Sprünge können eh nicht
      | kompensiert werden, da
      | Ventildynamik zu langsam
  Terminator2 : Terminator
  entl : Gain  Gain=-1
  offset [Pa] : Constant  Value=0.01  SampleTime=tA
      settings: AttributesFormatString=|
      | Num. Offset
      | ca. 0.01 Pa als numerische Begrenzung, dass
      | Ventildruck immer innerhalb der Druckbegrenzung
      | 
      | sample time: %<SampleTime>
  pValve-Filt : libc_filters_diff/PT1_konsistent
  switch : ManualSwitch
      settings: AttributesFormatString=|
      | Treibender Druck
      | gesättigt/gefiltert
      | oder nicht?
  u : Outport
  wires:
  switch/1 -> PsiPCmax_bel2/2
  offset [Pa]/1 -> Sum/2, Sum2/1
  Sum2/1 -> Saturation Dynamic/3
  Sum/1 -> Saturation Dynamic/1
  pH/1 -> Reine Durchflussfunktion 2-Kanal (sim)/1, PsiPCmax_bel1/2, Sum/1
  Saturation Dynamic/1 -> Reine Durchflussfunktion 2-Kanal (sim)/2, switch/1
  pL/1 -> Sum2/2, Reine Durchflussfunktion 2-Kanal (sim)/3
  Saturation Stellgroesse3/1 -> Leitwert (erweitert) (ent)/1
  Saturation Stellgroesse1/1 -> Leitwert (erweitert) (bel)/1
  Saturation Stellgroesse5/1 -> Sum1/2
  Leitwert (erweitert) (bel)/1 -> Saturation Stellgroesse4/1
  Demux/1 -> Leitwert (erweitert) (ent)/2
  Demux/2 -> Leitwert (erweitert) (ent)/3
  Demux/3 -> Leitwert (erweitert) (ent)/4
  Demux/4 -> Leitwert (erweitert) (ent)/5
  Demux/5 -> Leitwert (erweitert) (ent)/6
  Demux1/1 -> Leitwert (erweitert) (bel)/2
  Demux1/2 -> Leitwert (erweitert) (bel)/3
  Demux1/3 -> Leitwert (erweitert) (bel)/4
  Demux1/4 -> Leitwert (erweitert) (bel)/5
  Demux1/5 -> Leitwert (erweitert) (bel)/6
  valve-data-red-bel/1 -> Demux1/1
  valve-data-ext-ent/1 -> Demux/1
  Saturation Stellgroesse7/1 -> Cnlin_ent x Psi_ent/2
  Cnlin_bel/1 -> Saturation Stellgroesse1/1
  Cnlin_ent/1 -> Saturation Stellgroesse3/1
  pValve (Psi)/1 -> pValve-Filt/1, switch/2
  pValve-Filt/2 -> Terminator2/1
  T1_pValve/1 -> pValve-Filt/2
  pValve-Filt/1 -> Saturation Dynamic/2
  Saturation Stellgroesse6/1 -> Cnlin_bel x Psi_bel/2
  PsiPCmax_bel1/1 -> Cnlin_bel x Psi_bel/1
  PsiPCmax_bel2/1 -> Cnlin_ent x Psi_ent/1
  Cnlin_bel x Psi_bel/1 -> Cnlin_bel/1
  Psi_bel/1 -> Cnlin_bel/2
  Cnlin_ent x Psi_ent/1 -> entl/1
  Psi_ent/1 -> Cnlin_ent/2
  entl/1 -> Cnlin_ent/1
  dm_d/1 -> Saturation Stellgroesse6/1, Saturation Stellgroesse7/1
  rho/1 -> PsiPCmax_bel1/3, PsiPCmax_bel2/1
  Cmax-bel/1 -> PsiPCmax_bel1/1
  Cmax-ent/1 -> PsiPCmax_bel2/3
  Reine Durchflussfunktion 2-Kanal (sim)/2 -> Psi_ent/2
  Reine Durchflussfunktion 2-Kanal (sim)/1 -> Psi_bel/2
  b/1 -> Mux4/1, Mux4/2
  Mux4/1 -> Reine Durchflussfunktion 2-Kanal (sim)/4
  PsiMax/1 -> Psi_ent/1, Psi_bel/1
  Psi_min/1 -> Psi_bel/3, Psi_ent/3
  Leitwert (erweitert) (ent)/1 -> Saturation Stellgroesse5/1
  Demux/6 -> Leitwert (erweitert) (ent)/7
  Demux/7 -> Leitwert (erweitert) (ent)/8
  Demux/8 -> Leitwert (erweitert) (ent)/9
  Demux/9 -> Leitwert (erweitert) (ent)/10
  Demux/10 -> Leitwert (erweitert) (ent)/11
  Demux/11 -> Leitwert (erweitert) (ent)/12
  Demux1/6 -> Leitwert (erweitert) (bel)/7
  Demux1/7 -> Leitwert (erweitert) (bel)/8
  Demux1/8 -> Leitwert (erweitert) (bel)/9
  Demux1/9 -> Leitwert (erweitert) (bel)/10
  Demux1/10 -> Leitwert (erweitert) (bel)/11
  Demux1/11 -> Leitwert (erweitert) (bel)/12
  Saturation Stellgroesse4/1 -> Sum1/1
  Sum1/1 -> u/1

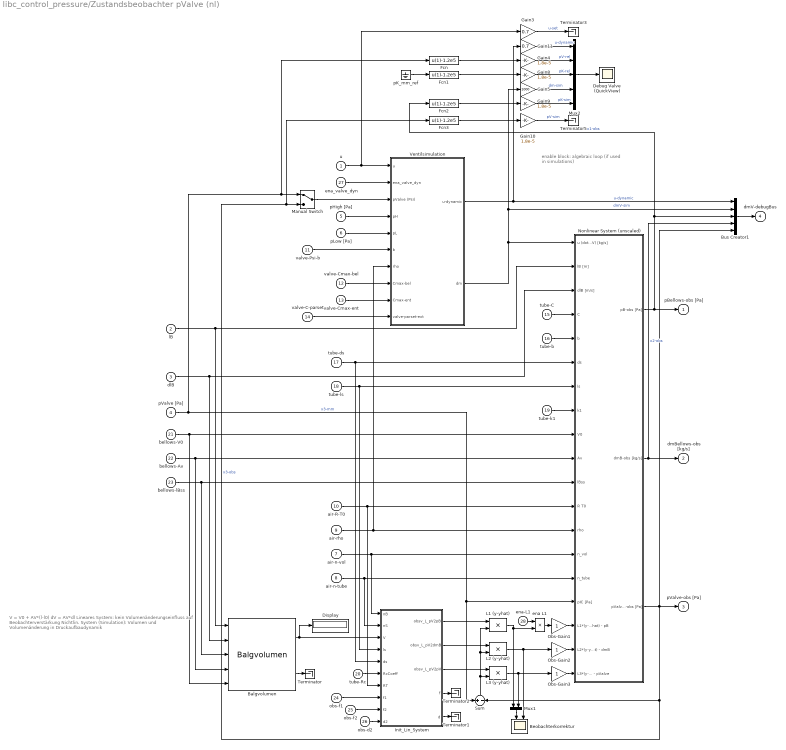
== system libc_control_pressure/Zustandsbeobachter pValve (nl) ==
  note: enable block:
      | algebraic loop
      | (if used in simulations)
  note: V = V0 + AV*(l-l0)
      | dV = AV*dl
      |
      | Lineares System:
      | kein Volumenänderungseinfluss auf Beobachterverstärkung
      |
      | Nichtlin. System (Simulation):
      | Volumen und Volumenänderung in Druckaufbaudynamik
  u : Inport
  lB : Inport  Port=2
  dlB : Inport  Port=3
  pValve [Pa] : Inport  Port=4
  pHigh [Pa] : Inport  Port=5
  pLow [Pa] : Inport  Port=6
  air-n-vol : Inport  Port=7
  air-n-tube : Inport  Port=8
  air-rho : Inport  Port=9
  air-R-T0 : Inport  Port=10
  valve-Psi-b : Inport  Port=11
  valve-Cmax-bel : Inport  Port=12
  valve-Cmax-ent : Inport  Port=13
  valve-C-parset : Inport  Port=14
  tube-C : Inport  Port=15
  tube-b : Inport  Port=16
  tube-ds : Inport  Port=17
  tube-ls : Inport  Port=18
  tube-k1 : Inport  Port=19
  tube-Rc : Inport  Port=20
  bellows-V0 : Inport  Port=21
  bellows-Av : Inport  Port=22
  bellows-lBss : Inport  Port=23
  obs-f1 : Inport  Port=24
  obs-f2 : Inport  Port=25
  obs-d2 : Inport  Port=26
  ena_valve_dyn : Inport  Port=27
  ena-L1 : Inport  Port=28
  Balgvolumen : libbha_parts_bellows/Balgvolumen
  Beobachterkorrektur : Scope  NumInputPorts=2
  Bus Creator1 : BusCreator  Inputs=5
  Debug Valve (QuickView) : Scope
  Display : Display
  Fcn{,1..3} (4 alike) : Fcn  Expr=u(1)-1.2e5
  Gain{4,8..10} (4 alike) : Gain  Gain=1.8e-5
  Gain11 : Gain  Gain=0.7
  Gain3 : Gain  Gain=0.7
  Gain5 : Gain  Gain=1000
  Init_Lin_System : MATLAB Function  TreatAsAtomicUnit=on
  L1 (y-yhat) : Product
      settings: AttributesFormatString=sat: 0.1e5
  L2 (y-yhat) : Product
  L3 (y-yhat) : Product
  Manual Switch : ManualSwitch
  Mux1 : Mux  Inputs=2
  Mux2 : Mux  Inputs=5
  Nonlinear System (unscaled) : Subsystem
  Obs-Gain1 : Gain
  Obs-Gain2 : Gain
  Obs-Gain3 : Gain
  Sum : Sum  Inputs=+|-
  Terminator{,1..3,5} (5 alike) : Terminator
  Ventilsimulation : Subsystem
  ena L1 : Product
  pK_mm_ref : Ground
  pBellows-obs [Pa] : Outport  PortDimensions=1
  dmBellows-obs [kg/s] : Outport  Port=2  PortDimensions=1
  pValve-obs [Pa] : Outport  Port=3  PortDimensions=1
  dmV-debugBus : Outport  Port=4
  wires:
  Ventilsimulation/1(u-dynamic) -> Gain11/1, Bus Creator1/1  "u-dynamic"
  Obs-Gain1/1 -> Nonlinear System (unscaled)/17(L1*(y-yhat) - pB)
  Obs-Gain3/1 -> Nonlinear System (unscaled)/19(L3*(y-yhat) - pValve)
  Obs-Gain2/1 -> Nonlinear System (unscaled)/18(L2*(y-yhat) - dmB)
  Mux1/1 -> Beobachterkorrektur/1
  valve-Cmax-ent/1 -> Ventilsimulation/9(Cmax-ent)
  Gain11/1 -> Mux2/1  "u-dynamic"
  Manual Switch/1 -> Ventilsimulation/3(pValve (Psi))
  Gain10/1 -> Terminator5/1  "pV-sim"
  Fcn3/1 -> Gain10/1
  Fcn2/1 -> Gain9/1
  Gain9/1 -> Mux2/5  "pK-sim"
  Gain8/1 -> Mux2/3  "pK-rel"
  Fcn1/1 -> Gain8/1
  pK_mm_ref/1 -> Fcn1/1
  Mux2/1 -> Debug Valve (QuickView)/1
  Fcn/1 -> Gain4/1
  Gain5/1 -> Mux2/4  "dm-sim"
  Gain4/1 -> Mux2/2  "pV-rel"
  Gain3/1 -> Terminator3/1  "u-set"
  air-n-vol/1 -> Nonlinear System (unscaled)/14(n_vol), Init_Lin_System/1(nB)
  Ventilsimulation/2(dm) -> Nonlinear System (unscaled)/1(u (dotmV) [kg/s]), Gain5/1, Bus Creator1/2  "dmV-sim"
  Init_Lin_System/4(f) -> Terminator2/1
  Init_Lin_System/5(d) -> Terminator1/1
  valve-Psi-b/1 -> Ventilsimulation/6(b)
  obs-f2/1 -> Init_Lin_System/9(f2)
  obs-d2/1 -> Init_Lin_System/10(d2)
  obs-f1/1 -> Init_Lin_System/8(f1)
  pLow [Pa]/1 -> Ventilsimulation/5(pL)
  pHigh [Pa]/1 -> Ventilsimulation/4(pH)
  valve-C-parset/1 -> Ventilsimulation/10(valve-parset-ext)
  valve-Cmax-bel/1 -> Ventilsimulation/8(Cmax-bel)
  air-R-T0/1 -> Nonlinear System (unscaled)/12(R T0), Init_Lin_System/7(RT)
  air-rho/1 -> Ventilsimulation/7(rho), Nonlinear System (unscaled)/13(rho)
  u/1 -> Gain3/1, Ventilsimulation/1(u)
  tube-Rc/1 -> Init_Lin_System/6(RcCoeff)
  bellows-Av/1 -> Nonlinear System (unscaled)/10(Av), Balgvolumen/4
  dlB/1 -> Nonlinear System (unscaled)/3(dlB [m/s]), Balgvolumen/2
  Balgvolumen/2 -> Terminator/1
  Balgvolumen/1 -> Init_Lin_System/3(V), Display/1
  tube-ls/1 -> Nonlinear System (unscaled)/7(ls), Init_Lin_System/4(ls)
  bellows-lBss/1 -> Nonlinear System (unscaled)/11(lBss), Balgvolumen/3
  bellows-V0/1 -> Nonlinear System (unscaled)/9(V0), Balgvolumen/5
  air-n-tube/1 -> Nonlinear System (unscaled)/15(n_tube), Init_Lin_System/2(nS)
  tube-k1/1 -> Nonlinear System (unscaled)/8(k1)
  lB/1 -> Nonlinear System (unscaled)/2(lB [m]), Balgvolumen/1
  tube-b/1 -> Nonlinear System (unscaled)/5(b)
  Init_Lin_System/1(obsv_L_pV2pB) -> L1 (y-yhat)/1
  Init_Lin_System/3(obsv_L_pV2pV) -> L3 (y-yhat)/1
  Init_Lin_System/2(obsv_L_pV2dmB) -> L2 (y-yhat)/1
  L3 (y-yhat)/1 -> Obs-Gain3/1, Mux1/2
  L2 (y-yhat)/1 -> Obs-Gain2/1, Beobachterkorrektur/2
  Nonlinear System (unscaled)/2(dmB-obs [kg/s]) -> Bus Creator1/4, dmBellows-obs [kg/s]/1  "x2-obs"
  Nonlinear System (unscaled)/1(pB-obs [Pa]) -> pBellows-obs [Pa]/1, Fcn2/1, Bus Creator1/3  "x1-obs"
  Nonlinear System (unscaled)/3(pValve-obs [Pa]) -> Sum/2, Fcn3/1, Manual Switch/2, Bus Creator1/5, pValve-obs [Pa]/1  "x3-obs"
  Sum/1 -> L3 (y-yhat)/2, L1 (y-yhat)/2, L2 (y-yhat)/2
  L1 (y-yhat)/1 -> ena L1/2, Mux1/1
  pValve [Pa]/1 -> Fcn/1, Manual Switch/1, Nonlinear System (unscaled)/16(pIC [Pa]), Sum/1  "x3-mm"
  tube-C/1 -> Nonlinear System (unscaled)/4(C)
  tube-ds/1 -> Nonlinear System (unscaled)/6(ds), Init_Lin_System/5(ds)
  Bus Creator1/1 -> dmV-debugBus/1
  ena_valve_dyn/1 -> Ventilsimulation/2(ena_valve_dyn)
  ena L1/1 -> Obs-Gain1/1
  ena-L1/1 -> ena L1/1
